simulink model "AMR_main_23b"  (R2024a)
settings: configuration reference "Configuration" (kept outside this file)
model workspace (MAT data in the model file):
  RTK_health_condition = 30
  mdlWSDbList = ["C:\Users\matlab.cut\Desktop\AMR\canbus_files\tramontina_database_nvidia.dbc" "C:\Users\matlab.cut\Desktop\AMR\canbus_files\tramontina_database_sick_modbus.dbc" "C:\Users\matlab.cut\Desktop\AMR\canbus_files\tramontina_database_xsens.dbc" "tramontina_database_curtis.dbc"]
undefined symbols (not defined in the file or in its folder): Down, Pull
libraries: speedgoatlib_IO60X_IO69X x17, tramontina_database_nvidialib x11, tramontina_database_curtislib x7, tramontina_database_xsenslib x4, tramontina_database_moboticlib x4, speedgoatlib_IO691 x3, canmsglib x2, slrealtimeseriallib x2, etargetslib x1, tramontina_database_sick_modbuslib x1
(part 1 of 2)
settings Model: DataDictionary=configuration_dictionary.sldd  Creator=matlab.cut  LastModifiedBy=rodri
settings ConfigSetRef: SourceName=Configuration

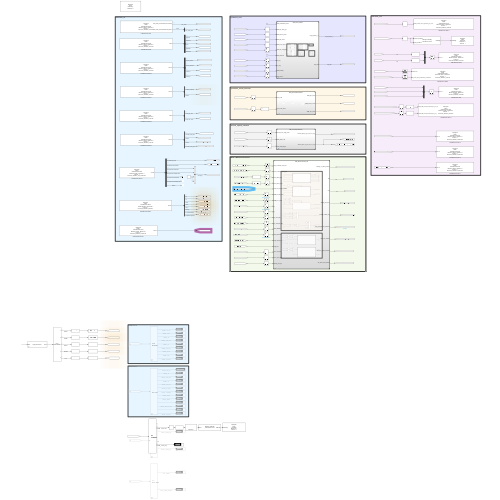
[thumbnail: Simulink's stored preview of the top-level diagram]
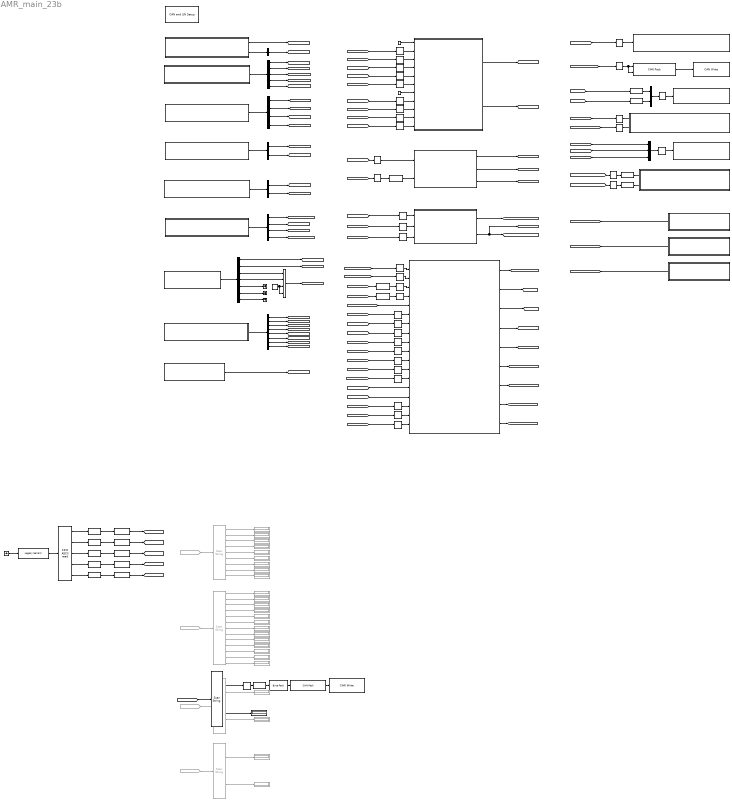
== system AMR_main_23b ==
  note: interface_in
  note: interface_out
  note: guidance_unit
  note: operation_mode_selector
  note: vehicle_speed_readout
  note: MCU - MotorControlUnit
  note: GPGGA Parser
  note: GPRMC Parser
  ASCII to String{,1..4} (5 alike) : ASCIIToString
  Bus Creator2 : BusCreator  Inputs=2
  Bus Creator3 : BusCreator  Inputs=3
  Bus Selector : BusSelector  OutputSignals=ID113_LongLat.latitude,ID113_LongLat.longitude,ID34_EulerAngles.yaw,ID17_StatusWord.GNSSfix,ID17_StatusWord.RtkStatus
  Bus Selector1 : BusSelector  OutputSignals=ID288_mobotic_feedback_pos.position_feedback,ID288_mobotic_feedback_pos.MessageStatus.Status
  Bus Selector2 : BusSelector  OutputSignals=ID422_curtis_feedback_message_left.motor_rpm_left,ID423_curtis_feedback_message_right.motor_rpm_right
  Bus Selector3 : BusSelector  OutputSignals=ID370_outdoor_scanner_PosX.X,ID371_outdoor_scanner_PosY.Y,ID372_outdoor_scanner_Yaw_Status.Yaw,ID373_outdoor_scanner_Odometer_Vel.velX,ID373_outdoor_scanner_Odometer_Vel.velY,ID373_outdoor_scanner_Odometer_Vel.velAng,ID372_outdoor_scanner_Yaw_Status.LocalizationStatus,ID372_outdoor_scanner_Yaw_Status.MapMatchingStatus
  Bus Selector4 : BusSelector  OutputSignals=Status  OutputAsBus=on
  Bus Selector5 : BusSelector  OutputSignals=ID368_joystick_axes.joystick_throttle,ID368_joystick_axes.joystick_direction,ID369_joystick_buttons.button_5,ID369_joystick_buttons.button_6
  Bus Selector6 : BusSelector  OutputSignals=ID1830_controller_status_left.controller_mode_left,ID1830_controller_status_left.MessageStatus.Status,ID1831_controller_status_right.MessageStatus.Status,ID1831_controller_status_right.controller_mode_right
  Bus Selector7 : BusSelector  OutputSignals=ID341_read_from_flexisoft.AuxEmEmergencia,ID341_read_from_flexisoft.AuxScannerInterrompido,ID341_read_from_flexisoft.EmergenciaFrontalDireita,ID341_read_from_flexisoft.EmergenciaFrontalEsquerda,ID341_read_from_flexisoft.EmergenciaTraseiraDireita,ID341_read_from_flexisoft.EmergenciaTraseiraEsquerda,ID341_read_from_flexisoft.MessageStatus.Status
  Byte Pack : etargetslib/Byte Pack  datatypes={'double'}  byteAlign=1
  CAN DB Parser Read : Subsystem
      settings: OpenFcn=sg_can.OpenFcnRead;
      mask Help: eval('sg.utils.help.show(''io_main/refentry_ref_can_ofa_parsing_read'');')
      mask Display: disp('Speedgoat\nIO691\nCAN DB Parser Read\nModule ID: IO691 - Module ID 1\nChannel:  1\ntramontina_database_xsens.dbc ');
  "CAN DB Parser Read " : Subsystem
      settings: OpenFcn=sg_can.OpenFcnRead;
      mask Help: eval('sg.utils.help.show(''io_main/refentry_ref_can_ofa_parsing_read'');')
      mask Display: disp('Speedgoat\nIO691\nCAN DB Parser Read\nModule ID: IO691 - Module ID 1\nChannel:  1\ntramontina_database_nvidia.dbc ');
  CAN DB Parser Read 1 : Subsystem
      settings: OpenFcn=sg_can.OpenFcnRead;
      mask Help: eval('sg.utils.help.show(''io_main/refentry_ref_can_ofa_parsing_read'');')
      mask Display: disp('Speedgoat\nIO691\nCAN DB Parser Read\nModule ID: IO691 - Module ID 1\nChannel:  1\ntramontina_database_nvidia.dbc ');
  CAN DB Parser Read 2 : Subsystem
      settings: OpenFcn=sg_can.OpenFcnRead;
      mask Help: eval('sg.utils.help.show(''io_main/refentry_ref_can_ofa_parsing_read'');')
      mask Display: disp('Speedgoat\nIO691\nCAN DB Parser Read\nModule ID: IO691 - Module ID 1\nChannel:  1\ntramontina_database_curtis.dbc ');
  CAN DB Parser Read 3 : Subsystem
      settings: OpenFcn=sg_can.OpenFcnRead;
      mask Help: eval('sg.utils.help.show(''io_main/refentry_ref_can_ofa_parsing_read'');')
      mask Display: disp('Speedgoat\nIO691\nCAN DB Parser Read\nModule ID: IO691 - Module ID 1\nChannel:  1\ntramontina_database_curtis.dbc ');
  CAN DB Parser Read 4 : Subsystem
      settings: OpenFcn=sg_can.OpenFcnRead;
      mask Help: eval('sg.utils.help.show(''io_main/refentry_ref_can_ofa_parsing_read'');')
      mask Display: disp('Speedgoat\nIO691\nCAN DB Parser Read\nModule ID: IO691 - Module ID 1\nChannel:  1\ntramontina_database_sick_modbus.dbc ');
  CAN DB Parser Read 5 : Subsystem
      settings: OpenFcn=sg_can.OpenFcnRead;
      mask Help: eval('sg.utils.help.show(''io_main/refentry_ref_can_ofa_parsing_read'');')
      mask Display: disp('Speedgoat\nIO691\nCAN DB Parser Read\nModule ID: IO691 - Module ID 1\nChannel:  1\ntramontina_database_nvidia.dbc ');
  CAN DB Parser Read 6 : Subsystem
      settings: OpenFcn=sg_can.OpenFcnRead;
      mask Help: eval('sg.utils.help.show(''io_main/refentry_ref_can_ofa_parsing_read'');')
      mask Display: disp('Speedgoat\nIO691\nCAN DB Parser Read\nModule ID: IO691 - Module ID 1\nChannel:  1\ntramontina_database_nvidia.dbc ');
  CAN DB Parser Read 7 : Subsystem
      settings: OpenFcn=sg_can.OpenFcnRead;
      mask Help: eval('sg.utils.help.show(''io_main/refentry_ref_can_ofa_parsing_read'');')
      mask Display: disp('Speedgoat\nIO691\nCAN DB Parser Read\nModule ID: IO691 - Module ID 1\nChannel:  1\ntramontina_database_mobotic.dbc ');
  "CAN DB Parser Write " : Subsystem
      settings: OpenFcn=sg_can.OpenFcnWrite;
      mask Help: eval('sg.utils.help.show(''io_main/refentry_ref_can_ofa_parsing_write'');')
      mask Display: disp('Speedgoat\nIO691\nCAN DB Parser Write\nModule ID: IO691 - Module ID 1\nChannel:  1\ntramontina_database_nvidia.dbc ');
  CAN DB Parser Write 1 : Subsystem
      settings: OpenFcn=sg_can.OpenFcnWrite;
      mask Help: eval('sg.utils.help.show(''io_main/refentry_ref_can_ofa_parsing_write'');')
      mask Display: disp('Speedgoat\nIO691\nCAN DB Parser Write\nModule ID: IO691 - Module ID 1\nChannel:  1\ntramontina_database_nvidia.dbc ');
  CAN DB Parser Write 2 : Subsystem
      settings: OpenFcn=sg_can.OpenFcnWrite;
      mask Help: eval('sg.utils.help.show(''io_main/refentry_ref_can_ofa_parsing_write'');')
      mask Display: disp('Speedgoat\nIO691\nCAN DB Parser Write\nModule ID: IO691 - Module ID 1\nChannel:  1\ntramontina_database_curtis.dbc ');
  CAN DB Parser Write 3 : Subsystem
      settings: OpenFcn=sg_can.OpenFcnWrite;
      mask Help: eval('sg.utils.help.show(''io_main/refentry_ref_can_ofa_parsing_write'');')
      mask Display: disp('Speedgoat\nIO691\nCAN DB Parser Write\nModule ID: IO691 - Module ID 1\nChannel:  1\ntramontina_database_curtis.dbc ');
  CAN DB Parser Write 4 : Subsystem
      settings: OpenFcn=sg_can.OpenFcnWrite;
      mask Help: eval('sg.utils.help.show(''io_main/refentry_ref_can_ofa_parsing_write'');')
      mask Display: disp('Speedgoat\nIO691\nCAN DB Parser Write\nModule ID: IO691 - Module ID 1\nChannel:  1\ntramontina_database_mobotic.dbc ');
  CAN DB Parser Write 5 : Subsystem
      settings: OpenFcn=sg_can.OpenFcnWrite;
      mask Help: eval('sg.utils.help.show(''io_main/refentry_ref_can_ofa_parsing_write'');')
      mask Display: disp('Speedgoat\nIO691\nCAN DB Parser Write\nModule ID: IO691 - Module ID 1\nChannel:  1\ntramontina_database_nvidia.dbc ');
  CAN DB Parser Write 6 : Subsystem
      settings: OpenFcn=sg_can.OpenFcnWrite;
      mask Help: eval('sg.utils.help.show(''io_main/refentry_ref_can_ofa_parsing_write'');')
      mask Display: disp('Speedgoat\nIO691\nCAN DB Parser Write\nModule ID: IO691 - Module ID 1\nChannel:  1\ntramontina_database_mobotic.dbc ');
  CAN DB Parser Write 7 : Subsystem
      settings: OpenFcn=sg_can.OpenFcnWrite;
      mask Help: eval('sg.utils.help.show(''io_main/refentry_ref_can_ofa_parsing_write'');')
      mask Display: disp('Speedgoat\nIO691\nCAN DB Parser Write\nModule ID: IO691 - Module ID 1\nChannel:  1\ntramontina_database_mobotic.dbc ');
  CAN Pack : canmsglib/CAN Pack  MsgList=(none)  MsgName=CAN Msg  MsgIDType=Standard (11-bit identifier)  MsgIdentifier=0x123  MsgLength=8  Remote=off  ApplyMinMax=off  BusOutput=on  SignalInfo={}
      settings: LibrarySourceBlock=embeddedtargetslib/Host Communication/CAN Pack  DataFormat=raw data
  CAN Pack2 : canmsglib/CAN Pack  MsgList=(none)  MsgName=CAN Msg  MsgIDType=Standard (11-bit identifier)  MsgIdentifier=0x120  MsgLength=8  Remote=off  ApplyMinMax=off  BusOutput=on  SignalInfo={ 'position_feedback', '0', '32', 'LE', 'signed', 'Standard', '0', '1', '0', '-inf', 'inf'; 'pulse_feedback', '32', '32', 'LE', 'signed', 'Standard', '0', '1', '0', '-Inf', 'Inf' }
      settings: DataFormat=manually specified signals
  CAN Write 1 : speedgoatlib_IO691/CAN Write   moduleType=IO691  id=1  channel=1  canType=CAN (HS)  messageType=CAN (HS)  useBusIn=on  numOfMsg=1  enableInput=off  enableStatusPort=off  ts=100e-3  initValues=[691 1 0.1 0 1 1 0 1 0 1]
      settings: SourceProductName=IO691
  CAN Write 2 : speedgoatlib_IO691/CAN Write   moduleType=IO691  id=1  channel=1  canType=CAN (HS)  messageType=CAN (HS)  useBusIn=on  numOfMsg=1  enableInput=off  enableStatusPort=off  ts=20e-3  initValues=[691 1 0.02 0 1 1 0 1 0 1]
      settings: SourceProductName=IO691
  "CAN and LIN Setup " : speedgoatlib_IO691/CAN and LIN Setup   moduleInitValues="[691    1    1   -1   -1]"  id=1  moduleType=IO691  pciSlot=-1  canChn1=CAN (HS)  canChn2=Disabled  canChn3=Disabled  canChn4=Disabled  linChn1=Disabled  linChn2=Disabled  canInitStructArray=[]  canTermStructArray=[]  gpioChnx=Disabled  canChn1InitValues="[2   2   8   1  16   3  19   2   2   5   2   0]"  arbBdrChn1=500 kBaud  clockDividerChn1=Enable  arbManBdrChn1=[8,1,16,3]  fdBdrChn1=5.0 MBaud  fdManBdrChn1=[2,2,5,2]  termResistor1=off  canChn2InitValues="[1   0   2   8  31   8  19   2   2   5   2   0]"  arbBdrChn2=1.0 MBaud  clockDividerChn2=Enable  arbManBdrChn2=[2,8,31,8]  fdBdrChn2=5.0 MBaud  fdManBdrChn2=[2,2,5,2]  termResistor2=off  canChn3InitValues="[1   0   2   8  31   8  19   2   2   5   2   0]"  arbBdrChn3=1.0 MBaud  clockDividerChn3=Enable  arbManBdrChn3=[2,8,31,8]  fdBdrChn3=5.0 MBaud  fdManBdrChn3=[2,2,5,2]  termResistor3=off  canChn4InitValues="[1   0   2   8  31   8  19   2   2   5   2   0]"  arbBdrChn4=1.0 MBaud  clockDividerChn4=Enable  arbManBdrChn4=[2,8,31,8]  fdBdrChn4=5.0 MBaud  fdManBdrChn4=[2,2,5,2]  termResistor4=off  linChn1InitValues="[0  9600]"  linBtrChn1=9600  linChn2InitValues="[0  9600]"  linBtrChn2=9600  doInitTermStruct="[0  5  0  0  0]"  parDoChannels=[1 2]  parDoVoltage=5  parDoInitValues=0  parDoReset=1  parNumOfDoS=0  parDiChannels=[3 4]  parDiVoltage=5  parDiPull=Pull-Down
      settings: LibrarySourceBlock=speedgoatlib_IO602_IO691/CAN and LIN Setup
  Cast{,6..9} (5 alike) : DataTypeConversion  OutDataTypeStr=uint8  SaturateOnIntegerOverflow=off  RndMeth=Floor
  Cast1 : DataTypeConversion  OutDataTypeStr=boolean  SaturateOnIntegerOverflow=off  RndMeth=Floor
  Cast10 : DataTypeConversion  OutDataTypeStr=double  SaturateOnIntegerOverflow=off  RndMeth=Floor
  Cast11 : DataTypeConversion  OutDataTypeStr=double  SaturateOnIntegerOverflow=off  RndMeth=Floor
  Cast12 : DataTypeConversion  OutDataTypeStr=double  SaturateOnIntegerOverflow=off  RndMeth=Floor
  Cast2 : DataTypeConversion  OutDataTypeStr=single  SaturateOnIntegerOverflow=off  RndMeth=Floor
  Cast3 : DataTypeConversion  OutDataTypeStr=single  SaturateOnIntegerOverflow=off  RndMeth=Floor
  Cast4 : DataTypeConversion  OutDataTypeStr=boolean  SaturateOnIntegerOverflow=off  RndMeth=Floor
  Cast5 : DataTypeConversion  OutDataTypeStr=boolean  SaturateOnIntegerOverflow=off  RndMeth=Floor
  Display{2..4,6,8..12,14..18,20..31} (26 alike) : Display  Commented=on
  Display5 : Display
  FIFO ASCII read : slrealtimeseriallib/FIFO ASCII read  header={'$GPGGA', '$GPRMC','$HEHDT','$HCHDM','$PTCF'}  term=[13 10]  hold=Hold last output if no new data  enable=off  maxsize=1024  outputtype=8 bit uint null terminated  sampletime=-1
  From18 : From  Commented=on  GotoTag=PTCF_decode
  From22 : From  Commented=on  GotoTag=GPRMC_decode
  From23 : From  Commented=on  GotoTag=GPGGA_decode
  From30 : From  Commented=on  GotoTag=HEHDT_decode
  Ground3 : Ground
  Legacy Serial F2 : slrealtimeseriallib/Mainboard/Legacy Serial F  port=Legacy Serial Port 1  baud=115200  width=8  nstop=1  parity=None  ctsmode=off  fifosize=1024  idtype=8 bit uint null terminated  sampletime=10e-3
  Model : ModelReference  ModelNameDialog=deployAGV_stateflow.slx  SimulationMode=Normal  ModelReferenceVersion=3.4
  Model1 : ModelReference  ModelNameDialog=AMR_OperationModeSelector.slx  SimulationMode=Normal  ModelReferenceVersion=2.0
  Model3 : ModelReference  ModelNameDialog=AMR_VehicleSpeedReadout.slx  SimulationMode=Normal  ModelReferenceVersion=2.0
  Model4 : ModelReference  ModelNameDialog=AMR_MotorControlUnit_23b.slx  SimulationMode=Normal  ModelReferenceVersion=2.3
  OR : Logic  Operator=OR  Inputs=4  AllPortsSameDT=off  OutDataTypeStr=boolean
  Rate Transition{,1..10,13..16,22..24,26,28..30,32..44} (35 alike) : RateTransition
  Rate Transition11 : RateTransition  OutPortSampleTimeOpt=Inherit
  Rate Transition12 : RateTransition  Deterministic=off
  Rate Transition21 : RateTransition  OutPortSampleTimeOpt=Inherit
  String to Double : ScanString  Commented=on  Format="\"$GPRMC,%f,%c,%f,%c,%f,%c,%f,,%d,,,%s\""
  String to Double1 : ScanString  Commented=on  Format="\"$GPGGA,%f,%f,%c,%f,%c,%d,%d,%f,%f,%c,%g,%c,,%f\""
  String to Double2 : ScanString  Commented=on  Format="\"$HEHDT,%f,%c\""
  String to Double3 : ScanString  Format="\"$HCHDM,%f,%c\""
  String to Double4 : ScanString  Commented=on  Format="\"$PTCF,%f,%c\""
  Terminator : Terminator
  Terminator1 : Terminator
  Terminator2 : Terminator
  Zero : Constant  Value=0  OutDataTypeStr=Inherit: Inherit via back propagation
  Zero1 : Constant  Value=0  OutDataTypeStr=Inherit: Inherit via back propagation
  Zero2 : Constant  Value=0  OutDataTypeStr=Inherit: Inherit via back propagation
  wires:
  Bus Selector7/2 -> [scanner_blocked]  "<AuxScannerInterrompido>"
  Bus Selector4/1 -> [oper_mode_status]  "oper_mode_status"
  Bus Selector6/4 -> [curtis_controller_mode_right]  "<controller_mode_right>"
  Bus Selector7/3 -> OR/1  "<EmergenciaFrontalDireita>"
  "CAN DB Parser Read "/1(ID343_AMR_OperationMode.OperationMode) -> [oper_mode]  "oper_mode"
  Bus Selector1/2 -> [steering_unit_status]  "<Status>"
  Bus Selector/1 -> [lat_deg]  "<latitude>"
  Bus Selector5/3 -> [joy_boost_flag]  "<button_5>"
  CAN DB Parser Read/1(CAN Rx) -> Bus Selector/1
  Bus Selector/5 -> [GPS_RTKstatus]  "<RtkStatus>"
  Bus Selector5/1 -> [xj]  "<joystick_throttle>"
  Zero/1 -> OR/3, OR/4
  Bus Selector/4 -> [GPS_GNSSfix]  "<GNSSfix>"
  Bus Selector6/2 -> [curtis_status_left]  "<Status>"
  Bus Selector/2 -> [lon_deg]  "<longitude>"
  Bus Selector7/6 -> Terminator1/1  "<EmergenciaTraseiraEsquerda>"
  "CAN DB Parser Read "/2(ID343_AMR_OperationMode.MessageStatus) -> Bus Selector4/1  "status"
  Bus Selector7/4 -> OR/2  "<EmergenciaFrontalEsquerda>"
  Bus Selector7/7 -> Terminator/1  "<Status>"
  Bus Selector5/2 -> [yj]  "<joystick_direction>"
  CAN DB Parser Read 2/1(CAN Rx) -> Bus Selector2/1
  Bus Selector2/2 -> [motor_rpm_right]  "<motor_rpm_right>"
  CAN DB Parser Read 4/1(CAN Rx) -> Bus Selector7/1
  CAN DB Parser Read 3/1(CAN Rx) -> Bus Selector6/1
  Bus Selector6/1 -> [curtis_controller_mode_left]  "<controller_mode_left>"
  Bus Selector2/1 -> [motor_rpm_left]  "<motor_rpm_left>"
  Bus Selector6/3 -> [curtis_status_right]  "<Status>"
  Bus Selector1/1 -> [steering_unit_pos]  "<position_feedback>"
  CAN DB Parser Read 5/1(CAN Rx) -> Bus Selector5/1
  Bus Selector/3 -> [AMR_heading]  "<yaw>"
  CAN DB Parser Read 1/1(CAN Rx) -> Bus Selector1/1
  OR/1 -> [emergency]  "emergency"
  Bus Selector5/4 -> [joy_maxspeed_flag]  "<button_6>"
  Bus Selector7/5 -> Terminator2/1  "<EmergenciaTraseiraDireita>"
  Bus Selector7/1 -> [interlock]  "<AuxEmEmergencia>"
  Rate Transition32/1 -> CAN DB Parser Write 5/1(ID289_mobotic_error_flag.steering_unit_error)
  Rate Transition28/1 -> Cast2/1
  [AMR_speed_to_CAN_m_per_sec] -> Rate Transition29/1
  [AMR_speed_to_CAN_m_per_min] -> Rate Transition28/1
  CAN Pack2/1 -> CAN Write 2/1
  Bus Creator2/1 -> Rate Transition15/1
  [rws] -> Cast11/1  "rws"
  Cast10/1 -> Bus Creator2/1
  Rate Transition6/1 -> CAN DB Parser Write 3/2(ID0_curtis_input_operational.pre_operational)
  Bus Creator3/1 -> Rate Transition12/1
  [steering_unit_error] -> Rate Transition32/1
  Rate Transition10/1 -> CAN Pack2/2, CAN Pack2/1
  Rate Transition29/1 -> Cast3/1
  [curtis_controller_into_operation] -> Rate Transition6/1
  [lws] -> Cast10/1  "lws"
  Cast11/1 -> Bus Creator2/2
  [steering_unit_theta_position] -> Rate Transition10/1
  [controller_enable_flag] -> Rate Transition24/1
  Rate Transition15/1 -> CAN DB Parser Write 2/1(CAN Tx)
  Rate Transition24/1 -> CAN DB Parser Write 3/1(Enable Input)
  [AMR_heading] -> Rate Transition39/1
  [lon_deg] -> Rate Transition36/1
  [AMR_manual_mode] -> Rate Transition30/1
  [interlock] -> Rate Transition44/1
  [emergency] -> Rate Transition43/1
  [scanner_blocked] -> Rate Transition42/1
  [lat_deg] -> Rate Transition35/1
  [AMR_speed] -> Rate Transition37/1
  Rate Transition44/1 -> Model/2
  Zero1/1 -> Model/1
  Rate Transition30/1 -> Model/3
  Model/1 -> [target_speed_m_s]  "target_speed_m_s"
  Model/2 -> [angle_diff]  "angle_diff"
  [oper_mode] -> Rate Transition/1
  Cast4/1 -> Model1/2
  Model1/1 -> [AMR_idle_mode]
  Model1/2 -> [AMR_manual_mode]
  Model1/3 -> [AMR_auto_mode]
  [xj] -> Rate Transition3/1
  [joy_boost_flag] -> Rate Transition5/1
  [curtis_controller_mode_left] -> Rate Transition21/1
  Rate Transition22/1 -> Model4/3
  [yj] -> Rate Transition4/1
  Rate Transition21/1 -> Model4/1
  Rate Transition23/1 -> Model4/4
  Rate Transition11/1 -> Model4/2
  [joy_maxspeed_flag] -> Rate Transition7/1
  [AMR_manual_mode] -> Rate Transition16/1
  [curtis_status_right] -> Cast1/1
  [curtis_status_left] -> Cast5/1
  [curtis_controller_mode_right] -> Rate Transition11/1
  [AMR_auto_mode] -> Rate Transition33/1
  [motor_rpm_right] -> Rate Transition41/1
  [steering_unit_pos] -> Rate Transition38/1
  [motor_rpm_left] -> Rate Transition40/1
  Model3/1 -> [AMR_speed_to_CAN_m_per_min]
  Model3/2 -> [AMR_speed_to_CAN_m_per_sec], [AMR_speed]
  Rate Transition38/1 -> Model3/1
  Rate Transition41/1 -> Model3/3
  Rate Transition40/1 -> Model3/2
  Model4/1 -> [steering_unit_theta_position]
  Model4/3 -> [rws]  "rws"
  Model4/2 -> [lws]  "lws"
  [GPS_GNSSfix] -> Rate Transition34/1
  [motor_rpm_left] -> Rate Transition26/1
  [motor_rpm_right] -> Rate Transition9/1
  [steering_unit_pos] -> Rate Transition14/1
  Model4/4 -> [steering_unit_error]
  Model4/5 -> [controller_enable_flag]
  Model4/6 -> [curtis_controller_into_operation]
  [GPS_RTKstatus] -> Rate Transition8/1
  Cast2/1 -> CAN DB Parser Write 1/1(ID290_AMR_vehicle_speed.speed_m_per_min)
  Cast3/1 -> CAN DB Parser Write 1/2(ID290_AMR_vehicle_speed.speed_m_per_s)
  [oper_mode_status] -> Rate Transition1/1
  [AMR_idle_mode] -> Bus Creator3/1
  [AMR_auto_mode] -> Bus Creator3/3
  [AMR_manual_mode] -> Bus Creator3/2
  Cast5/1 -> Rate Transition22/1
  Cast1/1 -> Rate Transition23/1
  Rate Transition12/1 -> "CAN DB Parser Write "/1(CAN Tx)
  Rate Transition/1 -> Model1/1
  Rate Transition1/1 -> Cast4/1
  CAN DB Parser Read 6/1(CAN Rx) -> Bus Selector3/1
  Bus Selector3/6 -> [sick_vel_ang]  "<velAng>"
  Bus Selector3/1 -> [sick_x]  "<X>"
  Bus Selector3/4 -> [sick_velx]  "<velX>"
  Bus Selector3/2 -> [sick_y]  "<Y>"
  Bus Selector3/3 -> [sick_yaw]  "<Yaw>"
  Bus Selector3/5 -> [sick_vely]  "<velY>"
  Bus Selector3/7 -> [sick_loc_status]  "<LocalizationStatus>"
  Bus Selector3/8 -> [sick_map_matching]  "<MapMatchingStatus>"
  Legacy Serial F2/1 -> FIFO ASCII read/1
  FIFO ASCII read/5 -> Cast6/1  "PTCF"
  From18/1 -> String to Double4/1
  Cast6/1 -> ASCII to String4/1
  String to Double4/2 -> Display30/1  "PTCF__heading_TrueNorth"
  ASCII to String3/1 -> [HCHDM_decode]
  String to Double4/1 -> Display31/1  "PTCF__heading"
  FIFO ASCII read/2 -> Cast/1  "GPRMC"
  String to Double/5 -> Display21/1  "GPRMC__lon"
  String to Double2/2 -> Display12/1  "HEHDT__heading_type"
  String to Double1/13 -> Display29/1  "GPGGA__checksum"
  ASCII to String4/1 -> [PTCF_decode]
  String to Double1/5 -> Display15/1  "GPGGA__east_west"
  String to Double1/10 -> Display28/1
  ASCII to String2/1 -> [GPGGA_decode]
  Cast9/1 -> ASCII to String3/1
  String to Double2/1 -> Display6/1  "HEHDT__heading_deg"
  FIFO ASCII read/3 -> Cast8/1  "HEHDT"
  String to Double/7 -> Display3/1  "GPRMC__speed"
  FIFO ASCII read/4 -> Cast9/1  "HCHDM"
  From23/1 -> String to Double1/1
  String to Double1/11 -> Display24/1  "GPGGA__mean_sea_level"
  String to Double1/1 -> Display14/1  "GPGGA__time_utc"
  String to Double/2 -> Display22/1  "GPRMC__status"
  FIFO ASCII read/1 -> Cast7/1  "GPGGA"
  [HCHDM_decode] -> String to Double3/1
  Cast/1 -> ASCII to String/1
  String to Double1/8 -> Display26/1  "GPGGA__HDOP"
  String to Double/3 -> Display23/1  "GPRMC__lat"
  String to Double1/7 -> Display18/1  "GPGGA__#_satellites"
  String to Double/6 -> Display2/1  "GPRMC__east_west"
  From22/1 -> String to Double/1
  String to Double/4 -> Display11/1  "GPRMC__north_south"
  Cast8/1 -> ASCII to String1/1
  String to Double1/12 -> Display25/1
  String to Double/8 -> Display4/1  "GPRMC__date"
  ASCII to String/1 -> [GPRMC_decode]
  String to Double/1 -> Display20/1  "GPRMC__time_utc"
  String to Double/9 -> Display8/1  "GPRMC__checksum"
  ASCII to String1/1 -> [HEHDT_decode]
  String to Double1/6 -> Display10/1  "GPGGA__fix_quality"
  String to Double1/2 -> Display16/1  "GPGGA__lat"
  From30/1 -> String to Double2/1
  String to Double3/1 -> Rate Transition2/1  "HCHDM__heading_deg"
  String to Double1/3 -> Display17/1  "GPGGA__north_south"
  String to Double1/4 -> Display9/1  "GPGGA__lon"
  String to Double3/2 -> Display5/1  "HCHDM__heading_mag"
  Ground3/1 -> Legacy Serial F2/1
  String to Double1/9 -> Display27/1  "GPGGA__altitude"
  Cast7/1 -> ASCII to String2/1
  Rate Transition2/1 -> Cast12/1
  Cast12/1 -> Byte Pack/1
  CAN Pack/1 -> CAN Write 1/1
  Rate Transition39/1 -> Model/10
  Rate Transition37/1 -> Model/11
  Zero2/1 -> Model/7
  Rate Transition43/1 -> Model/6
  Rate Transition42/1 -> Model/5
  [AMR_idle_mode] -> Rate Transition13/1
  Rate Transition35/1 -> Model/8
  Rate Transition36/1 -> Model/9
  Rate Transition13/1 -> Model/4
  Byte Pack/1 -> CAN Pack/1
  CAN DB Parser Read 7/1(CAN Rx) -> [read_error_register_CANRx]
  [read_error_register_CANRx] -> Model4/5
  Rate Transition16/1 -> Model4/6
  Rate Transition33/1 -> Model4/7
  Rate Transition3/1 -> Model4/8
  Rate Transition4/1 -> Model4/9
  Rate Transition5/1 -> Model4/10
  Rate Transition7/1 -> Model4/11
  Rate Transition34/1 -> Model4/12
  Rate Transition8/1 -> Model4/13
  [target_speed_m_s] -> Model4/14
  [angle_diff] -> Model4/15
  Rate Transition26/1 -> Model4/16
  Rate Transition9/1 -> Model4/17
  Rate Transition14/1 -> Model4/18
  Model4/7 -> [clear_error_CANTx]
  Model4/8 -> [read_error_request_CANTx]
  Model4/9 -> [set_sevice_state_CANTx]
  [clear_error_CANTx] -> CAN DB Parser Write 6/1(CAN Tx)
  [read_error_request_CANTx] -> CAN DB Parser Write 4/1(CAN Tx)
  [set_sevice_state_CANTx] -> CAN DB Parser Write 7/1(CAN Tx)

== system AMR_main_23b/CAN DB Parser Read ==
  ReadSubsystem : Subsystem
  UnpackSubsystem : Subsystem
  CAN Rx : Outport
  wires:
  ReadSubsystem/1(Raw_Rx) -> UnpackSubsystem/1(Unpack_In)
  ReadSubsystem/2(Status_Rx) -> UnpackSubsystem/2(Status Inport)
  UnpackSubsystem/1(Unpack_Out) -> CAN Rx/1

== system AMR_main_23b/CAN DB Parser Read  ==
  ReadSubsystem : Subsystem
  SelectSignal_1_1 : BusSelector  OutputSignals=ID343_AMR_OperationMode.OperationMode
  SelectStatus_1 : BusSelector  OutputSignals=ID343_AMR_OperationMode.MessageStatus
  UnpackSubsystem : Subsystem
  ID343_AMR_OperationMode.OperationMode : Outport
  ID343_AMR_OperationMode.MessageStatus : Outport  Port=2
  wires:
  ReadSubsystem/1(Raw_Rx) -> UnpackSubsystem/1(Unpack_In)
  ReadSubsystem/2(Status_Rx) -> UnpackSubsystem/2(Status Inport)
  UnpackSubsystem/1(Unpack_Out) -> SelectSignal_1_1/1, SelectStatus_1/1
  SelectSignal_1_1/1 -> ID343_AMR_OperationMode.OperationMode/1  "<OperationMode>"
  SelectStatus_1/1 -> ID343_AMR_OperationMode.MessageStatus/1  "<MessageStatus>"

== system AMR_main_23b/CAN DB Parser Read 1 ==
  ReadSubsystem : Subsystem
  UnpackSubsystem : Subsystem
  CAN Rx : Outport
  wires:
  ReadSubsystem/1(Raw_Rx) -> UnpackSubsystem/1(Unpack_In)
  ReadSubsystem/2(Status_Rx) -> UnpackSubsystem/2(Status Inport)
  UnpackSubsystem/1(Unpack_Out) -> CAN Rx/1

== system AMR_main_23b/CAN DB Parser Read 2 ==
  ReadSubsystem : Subsystem
  UnpackSubsystem : Subsystem
  CAN Rx : Outport
  wires:
  ReadSubsystem/1(Raw_Rx) -> UnpackSubsystem/1(Unpack_In)
  ReadSubsystem/2(Status_Rx) -> UnpackSubsystem/2(Status Inport)
  UnpackSubsystem/1(Unpack_Out) -> CAN Rx/1

== system AMR_main_23b/CAN DB Parser Read 3 ==
  ReadSubsystem : Subsystem
  UnpackSubsystem : Subsystem
  CAN Rx : Outport
  wires:
  ReadSubsystem/1(Raw_Rx) -> UnpackSubsystem/1(Unpack_In)
  ReadSubsystem/2(Status_Rx) -> UnpackSubsystem/2(Status Inport)
  UnpackSubsystem/1(Unpack_Out) -> CAN Rx/1

== system AMR_main_23b/CAN DB Parser Read 4 ==
  ReadSubsystem : Subsystem
  UnpackSubsystem : Subsystem
  CAN Rx : Outport
  wires:
  ReadSubsystem/1(Raw_Rx) -> UnpackSubsystem/1(Unpack_In)
  ReadSubsystem/2(Status_Rx) -> UnpackSubsystem/2(Status Inport)
  UnpackSubsystem/1(Unpack_Out) -> CAN Rx/1

== system AMR_main_23b/CAN DB Parser Read 5 ==
  ReadSubsystem : Subsystem
  UnpackSubsystem : Subsystem
  CAN Rx : Outport
  wires:
  ReadSubsystem/1(Raw_Rx) -> UnpackSubsystem/1(Unpack_In)
  ReadSubsystem/2(Status_Rx) -> UnpackSubsystem/2(Status Inport)
  UnpackSubsystem/1(Unpack_Out) -> CAN Rx/1

== system AMR_main_23b/CAN DB Parser Read 6 ==
  ReadSubsystem : Subsystem
  UnpackSubsystem : Subsystem
  CAN Rx : Outport
  wires:
  ReadSubsystem/1(Raw_Rx) -> UnpackSubsystem/1(Unpack_In)
  ReadSubsystem/2(Status_Rx) -> UnpackSubsystem/2(Status Inport)
  UnpackSubsystem/1(Unpack_Out) -> CAN Rx/1

== system AMR_main_23b/CAN DB Parser Read 7 ==
  ReadSubsystem : Subsystem
  UnpackSubsystem : Subsystem
  CAN Rx : Outport
  wires:
  ReadSubsystem/1(Raw_Rx) -> UnpackSubsystem/1(Unpack_In)
  ReadSubsystem/2(Status_Rx) -> UnpackSubsystem/2(Status Inport)
  UnpackSubsystem/1(Unpack_Out) -> CAN Rx/1

== system AMR_main_23b/CAN DB Parser Write  ==
  CAN Tx : Inport
  BusMapping : Subsystem
  CANWrite : speedgoatlib_IO60X_IO69X/CAN/CAN Write   moduleType=IO691  id=1  channel=1  canType=CAN (HS)  messageType=CAN (HS)  useBusIn=on  numOfMsg=1  enableInput=on  enableStatusPort=off  ts=500e-3  initValues=[691 1 0.5 0 1 1 0 1 1 1]
  Convert2BusArray : Subsystem
  Enable All : Constant  OutDataTypeStr=boolean
  PackSubsystem : Subsystem
  Product : Product  OutDataTypeStr=uint32
  TxControl : Constant  Value=[1]  OutDataTypeStr=uint32
  wires:
  PackSubsystem/1(PackOut) -> Convert2BusArray/1(InBus)
  Convert2BusArray/1(BusArrayOut) -> CANWrite/2
  Product/1 -> CANWrite/1
  TxControl/1 -> Product/2
  Enable All/1 -> Product/1
  CAN Tx/1 -> BusMapping/1(InBus)
  BusMapping/1(OutBus) -> PackSubsystem/1(PackIn)

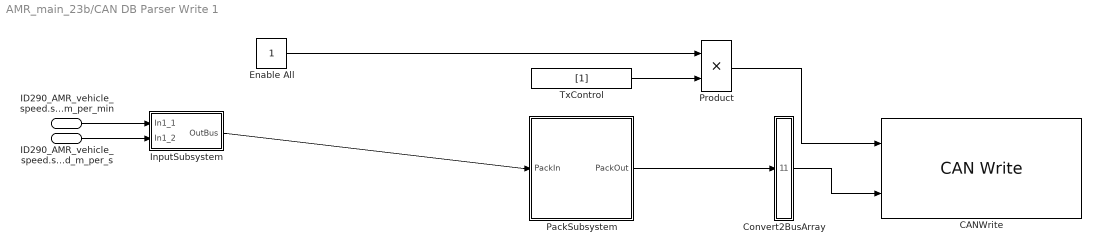
== system AMR_main_23b/CAN DB Parser Write 1 ==
  ID290_AMR_vehicle_speed.speed_m_per_min : Inport
  ID290_AMR_vehicle_speed.speed_m_per_s : Inport  Port=2
  CANWrite : speedgoatlib_IO60X_IO69X/CAN/CAN Write   moduleType=IO691  id=1  channel=1  canType=CAN (HS)  messageType=CAN (HS)  useBusIn=on  numOfMsg=1  enableInput=on  enableStatusPort=off  ts=50e-3  initValues=[691 1 0.05 0 1 1 0 1 1 1]
  Convert2BusArray : Subsystem
  Enable All : Constant  OutDataTypeStr=boolean
  InputSubsystem : Subsystem
  PackSubsystem : Subsystem
  Product : Product  OutDataTypeStr=uint32
  TxControl : Constant  Value=[1]  OutDataTypeStr=uint32
  wires:
  PackSubsystem/1(PackOut) -> Convert2BusArray/1(InBus)
  Convert2BusArray/1(BusArrayOut) -> CANWrite/2
  Product/1 -> CANWrite/1
  TxControl/1 -> Product/2
  Enable All/1 -> Product/1
  ID290_AMR_vehicle_speed.speed_m_per_min/1 -> InputSubsystem/1(In1_1)
  ID290_AMR_vehicle_speed.speed_m_per_s/1 -> InputSubsystem/2(In1_2)
  InputSubsystem/1(OutBus) -> PackSubsystem/1(PackIn)

== system AMR_main_23b/CAN DB Parser Write 2 ==
  CAN Tx : Inport
  BusMapping : Subsystem
  CANWrite : speedgoatlib_IO60X_IO69X/CAN/CAN Write   moduleType=IO691  id=1  channel=1  canType=CAN (HS)  messageType=CAN (HS)  useBusIn=on  numOfMsg=2  enableInput=on  enableStatusPort=off  ts=10e-3  initValues=[691 1 0.01 0 1 1 0 2 1 1]
  Convert2BusArray : Subsystem
  Enable All : Constant  OutDataTypeStr=boolean
  PackSubsystem : Subsystem
  Product : Product  OutDataTypeStr=uint32
  TxControl : Constant  Value="[1  1]"  OutDataTypeStr=uint32
  wires:
  PackSubsystem/1(PackOut) -> Convert2BusArray/1(InBus)
  Convert2BusArray/1(BusArrayOut) -> CANWrite/2
  Product/1 -> CANWrite/1
  TxControl/1 -> Product/2
  Enable All/1 -> Product/1
  CAN Tx/1 -> BusMapping/1(InBus)
  BusMapping/1(OutBus) -> PackSubsystem/1(PackIn)

== system AMR_main_23b/CAN DB Parser Write 3 ==
  Enable Input : Inport  OutDataTypeStr=boolean
  ID0_curtis_input_operational.pre_operational : Inport  Port=2
  CANWrite : speedgoatlib_IO60X_IO69X/CAN/CAN Write   moduleType=IO691  id=1  channel=1  canType=CAN (HS)  messageType=CAN (HS)  useBusIn=on  numOfMsg=1  enableInput=on  enableStatusPort=off  ts=500e-3  initValues=[691 1 0.5 0 1 1 0 1 1 1]
  Convert2BusArray : Subsystem
  InputSubsystem : Subsystem
  PackSubsystem : Subsystem
  Product : Product  OutDataTypeStr=uint32
  TxControl : Constant  Value=[1]  OutDataTypeStr=uint32
  wires:
  PackSubsystem/1(PackOut) -> Convert2BusArray/1(InBus)
  Convert2BusArray/1(BusArrayOut) -> CANWrite/2
  Product/1 -> CANWrite/1
  TxControl/1 -> Product/2
  Enable Input/1 -> Product/1
  ID0_curtis_input_operational.pre_operational/1 -> InputSubsystem/1(In1_1)
  InputSubsystem/1(OutBus) -> PackSubsystem/1(PackIn)

== system AMR_main_23b/CAN DB Parser Write 4 ==
  CAN Tx : Inport
  BusMapping : Subsystem
  CANWrite : speedgoatlib_IO60X_IO69X/CAN/CAN Write   moduleType=IO691  id=1  channel=1  canType=CAN (HS)  messageType=CAN (HS)  useBusIn=on  numOfMsg=1  enableInput=on  enableStatusPort=off  ts=-1  initValues=[691 1 -1 0 1 1 0 1 1 1]
  Convert2BusArray : Subsystem
  Enable All : Constant  OutDataTypeStr=boolean
  PackSubsystem : Subsystem
  Product : Product  OutDataTypeStr=uint32
  TxControl : Constant  Value=[1]  OutDataTypeStr=uint32
  wires:
  PackSubsystem/1(PackOut) -> Convert2BusArray/1(InBus)
  Convert2BusArray/1(BusArrayOut) -> CANWrite/2
  Product/1 -> CANWrite/1
  TxControl/1 -> Product/2
  Enable All/1 -> Product/1
  CAN Tx/1 -> BusMapping/1(InBus)
  BusMapping/1(OutBus) -> PackSubsystem/1(PackIn)

== system AMR_main_23b/CAN DB Parser Write 5 ==
  ID289_mobotic_error_flag.steering_unit_error : Inport
  CANWrite : speedgoatlib_IO60X_IO69X/CAN/CAN Write   moduleType=IO691  id=1  channel=1  canType=CAN (HS)  messageType=CAN (HS)  useBusIn=on  numOfMsg=1  enableInput=on  enableStatusPort=off  ts=500e-3  initValues=[691 1 0.5 0 1 1 0 1 1 1]
  Convert2BusArray : Subsystem
  Enable All : Constant  OutDataTypeStr=boolean
  InputSubsystem : Subsystem
  PackSubsystem : Subsystem
  Product : Product  OutDataTypeStr=uint32
  TxControl : Constant  Value=[1]  OutDataTypeStr=uint32
  wires:
  PackSubsystem/1(PackOut) -> Convert2BusArray/1(InBus)
  Convert2BusArray/1(BusArrayOut) -> CANWrite/2
  Product/1 -> CANWrite/1
  TxControl/1 -> Product/2
  Enable All/1 -> Product/1
  ID289_mobotic_error_flag.steering_unit_error/1 -> InputSubsystem/1(In1_1)
  InputSubsystem/1(OutBus) -> PackSubsystem/1(PackIn)

== system AMR_main_23b/CAN DB Parser Write 6 ==
  CAN Tx : Inport
  BusMapping : Subsystem
  CANWrite : speedgoatlib_IO60X_IO69X/CAN/CAN Write   moduleType=IO691  id=1  channel=1  canType=CAN (HS)  messageType=CAN (HS)  useBusIn=on  numOfMsg=1  enableInput=on  enableStatusPort=off  ts=-1  initValues=[691 1 -1 0 1 1 0 1 1 1]
  Convert2BusArray : Subsystem
  Enable All : Constant  OutDataTypeStr=boolean
  PackSubsystem : Subsystem
  Product : Product  OutDataTypeStr=uint32
  TxControl : Constant  Value=[1]  OutDataTypeStr=uint32
  wires:
  PackSubsystem/1(PackOut) -> Convert2BusArray/1(InBus)
  Convert2BusArray/1(BusArrayOut) -> CANWrite/2
  Product/1 -> CANWrite/1
  TxControl/1 -> Product/2
  Enable All/1 -> Product/1
  CAN Tx/1 -> BusMapping/1(InBus)
  BusMapping/1(OutBus) -> PackSubsystem/1(PackIn)

== system AMR_main_23b/CAN DB Parser Write 7 ==
  CAN Tx : Inport
  BusMapping : Subsystem
  CANWrite : speedgoatlib_IO60X_IO69X/CAN/CAN Write   moduleType=IO691  id=1  channel=1  canType=CAN (HS)  messageType=CAN (HS)  useBusIn=on  numOfMsg=1  enableInput=on  enableStatusPort=off  ts=-1  initValues=[691 1 -1 0 1 1 0 1 1 1]
  Convert2BusArray : Subsystem
  Enable All : Constant  OutDataTypeStr=boolean
  PackSubsystem : Subsystem
  Product : Product  OutDataTypeStr=uint32
  TxControl : Constant  Value=[1]  OutDataTypeStr=uint32
  wires:
  PackSubsystem/1(PackOut) -> Convert2BusArray/1(InBus)
  Convert2BusArray/1(BusArrayOut) -> CANWrite/2
  Product/1 -> CANWrite/1
  TxControl/1 -> Product/2
  Enable All/1 -> Product/1
  CAN Tx/1 -> BusMapping/1(InBus)
  BusMapping/1(OutBus) -> PackSubsystem/1(PackIn)

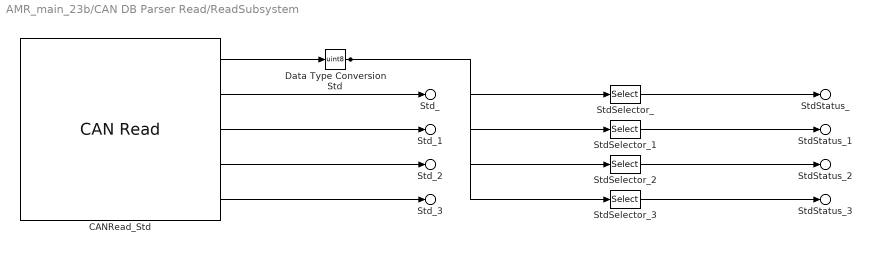
== system AMR_main_23b/CAN DB Parser Read/ReadSubsystem ==
  CANRead_Std : speedgoatlib_IO60X_IO69X/CAN/CAN Read   moduleType=IO691  id=1  channel=1  canType=CAN (HS)  messageType=CAN (HS)  useBusOut=on  HasMulRead=Specify by IDs  MsgIDlist="[17   34  113  118]"  isEFF=off  LabelInHex=off  enableInput=off  initValues=[691 1 0.005 0 1 1 0 1 2 0 4 17 34 113 118]  ts=5e-3
  Data Type ConversionStd : DataTypeConversion  OutDataTypeStr=uint8  SaturateOnIntegerOverflow=off  RndMeth=Floor
  StdSelector_ : Selector  IndexOptions=Index vector (dialog)  Indices=1  OutputSizes=1
  StdSelector_1 : Selector  IndexOptions=Index vector (dialog)  Indices=2  OutputSizes=1
  StdSelector_2 : Selector  IndexOptions=Index vector (dialog)  Indices=3  OutputSizes=1
  StdSelector_3 : Selector  IndexOptions=Index vector (dialog)  Indices=4  OutputSizes=1
  Std_ : Outport  PortName=Raw_Rx  Element=Std.ID17
  Std_1 : Outport  PortName=Raw_Rx  Element=Std.ID34
  Std_2 : Outport  PortName=Raw_Rx  Element=Std.ID113
  Std_3 : Outport  PortName=Raw_Rx  Element=Std.ID118
  StdStatus_ : Outport  Port=2  PortName=Status_Rx  Element=Std.ID17
  StdStatus_1 : Outport  Port=2  PortName=Status_Rx  Element=Std.ID34
  StdStatus_2 : Outport  Port=2  PortName=Status_Rx  Element=Std.ID113
  StdStatus_3 : Outport  Port=2  PortName=Status_Rx  Element=Std.ID118
  wires:
  CANRead_Std/1 -> Data Type ConversionStd/1
  CANRead_Std/2 -> Std_/1
  CANRead_Std/3 -> Std_1/1
  CANRead_Std/4 -> Std_2/1
  CANRead_Std/5 -> Std_3/1
  Data Type ConversionStd/1 -> StdSelector_/1, StdSelector_1/1, StdSelector_2/1, StdSelector_3/1
  StdSelector_/1 -> StdStatus_/1
  StdSelector_1/1 -> StdStatus_1/1
  StdSelector_2/1 -> StdStatus_2/1
  StdSelector_3/1 -> StdStatus_3/1

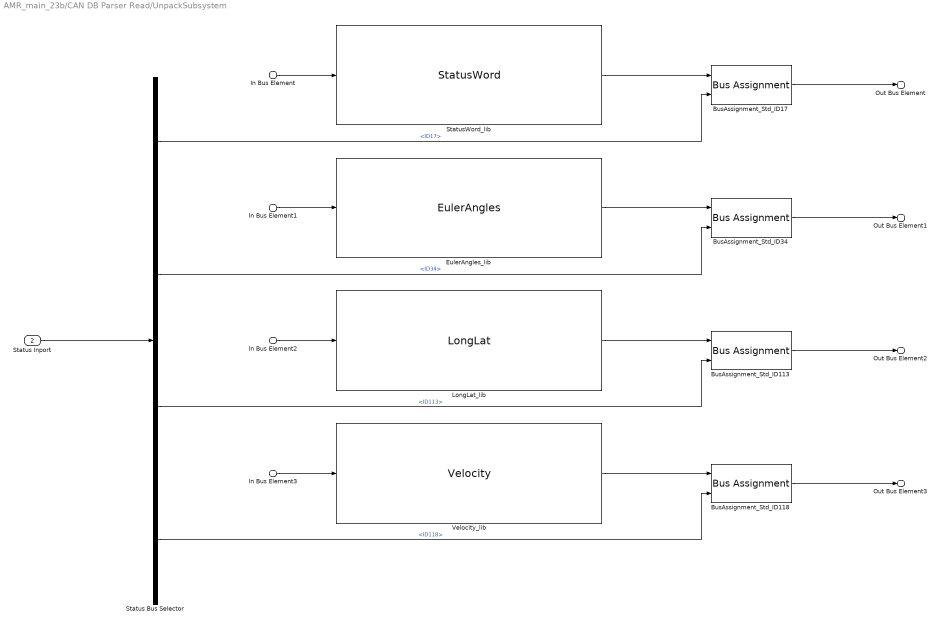
== system AMR_main_23b/CAN DB Parser Read/UnpackSubsystem ==
  In Bus Element : Inport  PortName=Unpack_In  Element=Std.ID17
  In Bus Element1 : Inport  PortName=Unpack_In  Element=Std.ID34
  In Bus Element2 : Inport  PortName=Unpack_In  Element=Std.ID113
  In Bus Element3 : Inport  PortName=Unpack_In  Element=Std.ID118
  Status Inport : Inport  Port=2
  BusAssignment_Std_ID{17,34,113,118} (4 alike) : BusAssignment  AssignedSignals=MessageStatus.Status
  EulerAngles_lib : tramontina_database_xsenslib/CAN unpack/EulerAngles  SystemSampleTime=-1  VariantActivationTime=update diagram  AllowFlexibleInterface=on  Latency=0  AutoFrameSizeCalculation=off
  LongLat_lib : tramontina_database_xsenslib/CAN unpack/LongLat  SystemSampleTime=-1  VariantActivationTime=update diagram  AllowFlexibleInterface=on  Latency=0  AutoFrameSizeCalculation=off
  Status Bus Selector : BusSelector  OutputSignals=Std.ID17,Std.ID34,Std.ID113,Std.ID118
  StatusWord_lib : tramontina_database_xsenslib/CAN unpack/StatusWord  SystemSampleTime=-1  VariantActivationTime=update diagram  AllowFlexibleInterface=on  Latency=0  AutoFrameSizeCalculation=off
  Velocity_lib : tramontina_database_xsenslib/CAN unpack/Velocity  SystemSampleTime=-1  VariantActivationTime=update diagram  AllowFlexibleInterface=on  Latency=0  AutoFrameSizeCalculation=off
  Out Bus Element : Outport  PortName=Unpack_Out  Element=ID17_StatusWord
  Out Bus Element1 : Outport  PortName=Unpack_Out  Element=ID34_EulerAngles
  Out Bus Element2 : Outport  PortName=Unpack_Out  Element=ID113_LongLat
  Out Bus Element3 : Outport  PortName=Unpack_Out  Element=ID118_Velocity
  wires:
  In Bus Element/1 -> StatusWord_lib/1
  StatusWord_lib/1 -> BusAssignment_Std_ID17/1
  BusAssignment_Std_ID17/1 -> Out Bus Element/1
  In Bus Element1/1 -> EulerAngles_lib/1
  EulerAngles_lib/1 -> BusAssignment_Std_ID34/1
  BusAssignment_Std_ID34/1 -> Out Bus Element1/1
  In Bus Element2/1 -> LongLat_lib/1
  LongLat_lib/1 -> BusAssignment_Std_ID113/1
  BusAssignment_Std_ID113/1 -> Out Bus Element2/1
  In Bus Element3/1 -> Velocity_lib/1
  Velocity_lib/1 -> BusAssignment_Std_ID118/1
  BusAssignment_Std_ID118/1 -> Out Bus Element3/1
  Status Inport/1 -> Status Bus Selector/1
  Status Bus Selector/1 -> BusAssignment_Std_ID17/2  "<ID17>"
  Status Bus Selector/2 -> BusAssignment_Std_ID34/2  "<ID34>"
  Status Bus Selector/3 -> BusAssignment_Std_ID113/2  "<ID113>"
  Status Bus Selector/4 -> BusAssignment_Std_ID118/2  "<ID118>"

== system AMR_main_23b/CAN DB Parser Read /ReadSubsystem ==
  CANRead_Std : speedgoatlib_IO60X_IO69X/CAN/CAN Read   moduleType=IO691  id=1  channel=1  canType=CAN (HS)  messageType=CAN (HS)  useBusOut=on  HasMulRead=Specify by IDs  MsgIDlist=[343]  isEFF=off  LabelInHex=off  enableInput=off  initValues=[691 1 0.05 0 1 1 0 1 2 0 1 343]  ts=50e-3
  Data Type ConversionStd : DataTypeConversion  OutDataTypeStr=uint8  SaturateOnIntegerOverflow=off  RndMeth=Floor
  StdSelector_ : Selector  IndexOptions=Index vector (dialog)  Indices=1  OutputSizes=1
  Std_ : Outport  PortName=Raw_Rx  Element=Std.ID343
  StdStatus_ : Outport  Port=2  PortName=Status_Rx  Element=Std.ID343
  wires:
  CANRead_Std/1 -> Data Type ConversionStd/1
  CANRead_Std/2 -> Std_/1
  Data Type ConversionStd/1 -> StdSelector_/1
  StdSelector_/1 -> StdStatus_/1

== system AMR_main_23b/CAN DB Parser Read /UnpackSubsystem ==
  In Bus Element : Inport  PortName=Unpack_In  Element=Std.ID343
  Status Inport : Inport  Port=2
  AMR_OperationMode_lib : tramontina_database_nvidialib/CAN unpack/AMR_OperationMode  SystemSampleTime=-1  VariantActivationTime=update diagram  AllowFlexibleInterface=on  Latency=0  AutoFrameSizeCalculation=off
  BusAssignment_Std_ID343 : BusAssignment  AssignedSignals=MessageStatus.Status
  Status Bus Selector : BusSelector  OutputSignals=Std.ID343
  Out Bus Element : Outport  PortName=Unpack_Out  Element=ID343_AMR_OperationMode
  wires:
  In Bus Element/1 -> AMR_OperationMode_lib/1
  AMR_OperationMode_lib/1 -> BusAssignment_Std_ID343/1
  BusAssignment_Std_ID343/1 -> Out Bus Element/1
  Status Inport/1 -> Status Bus Selector/1
  Status Bus Selector/1 -> BusAssignment_Std_ID343/2  "<ID343>"

== system AMR_main_23b/CAN DB Parser Read 1/ReadSubsystem ==
  CANRead_Std : speedgoatlib_IO60X_IO69X/CAN/CAN Read   moduleType=IO691  id=1  channel=1  canType=CAN (HS)  messageType=CAN (HS)  useBusOut=on  HasMulRead=Specify by IDs  MsgIDlist=[288]  isEFF=off  LabelInHex=off  enableInput=off  initValues=[691 1 0.005 0 1 1 0 1 2 0 1 288]  ts=5e-3
  Data Type ConversionStd : DataTypeConversion  OutDataTypeStr=uint8  SaturateOnIntegerOverflow=off  RndMeth=Floor
  StdSelector_ : Selector  IndexOptions=Index vector (dialog)  Indices=1  OutputSizes=1
  Std_ : Outport  PortName=Raw_Rx  Element=Std.ID288
  StdStatus_ : Outport  Port=2  PortName=Status_Rx  Element=Std.ID288
  wires:
  CANRead_Std/1 -> Data Type ConversionStd/1
  CANRead_Std/2 -> Std_/1
  Data Type ConversionStd/1 -> StdSelector_/1
  StdSelector_/1 -> StdStatus_/1

== system AMR_main_23b/CAN DB Parser Read 1/UnpackSubsystem ==
  In Bus Element : Inport  PortName=Unpack_In  Element=Std.ID288
  Status Inport : Inport  Port=2
  BusAssignment_Std_ID288 : BusAssignment  AssignedSignals=MessageStatus.Status
  Status Bus Selector : BusSelector  OutputSignals=Std.ID288
  mobotic_feedback_pos_lib : tramontina_database_nvidialib/CAN unpack/mobotic_feedback_pos  SystemSampleTime=-1  VariantActivationTime=update diagram  AllowFlexibleInterface=on  Latency=0  AutoFrameSizeCalculation=off
  Out Bus Element : Outport  PortName=Unpack_Out  Element=ID288_mobotic_feedback_pos
  wires:
  In Bus Element/1 -> mobotic_feedback_pos_lib/1
  mobotic_feedback_pos_lib/1 -> BusAssignment_Std_ID288/1
  BusAssignment_Std_ID288/1 -> Out Bus Element/1
  Status Inport/1 -> Status Bus Selector/1
  Status Bus Selector/1 -> BusAssignment_Std_ID288/2  "<ID288>"

== system AMR_main_23b/CAN DB Parser Read 2/ReadSubsystem ==
  CANRead_Std : speedgoatlib_IO60X_IO69X/CAN/CAN Read   moduleType=IO691  id=1  channel=1  canType=CAN (HS)  messageType=CAN (HS)  useBusOut=on  HasMulRead=Specify by IDs  MsgIDlist="[422  423]"  isEFF=off  LabelInHex=off  enableInput=off  initValues=[691 1 0.05 0 1 1 0 1 2 0 2 422 423]  ts=50e-3
  Data Type ConversionStd : DataTypeConversion  OutDataTypeStr=uint8  SaturateOnIntegerOverflow=off  RndMeth=Floor
  StdSelector_ : Selector  IndexOptions=Index vector (dialog)  Indices=1  OutputSizes=1
  StdSelector_1 : Selector  IndexOptions=Index vector (dialog)  Indices=2  OutputSizes=1
  Std_ : Outport  PortName=Raw_Rx  Element=Std.ID422
  Std_1 : Outport  PortName=Raw_Rx  Element=Std.ID423
  StdStatus_ : Outport  Port=2  PortName=Status_Rx  Element=Std.ID422
  StdStatus_1 : Outport  Port=2  PortName=Status_Rx  Element=Std.ID423
  wires:
  CANRead_Std/1 -> Data Type ConversionStd/1
  CANRead_Std/2 -> Std_/1
  CANRead_Std/3 -> Std_1/1
  Data Type ConversionStd/1 -> StdSelector_/1, StdSelector_1/1
  StdSelector_/1 -> StdStatus_/1
  StdSelector_1/1 -> StdStatus_1/1

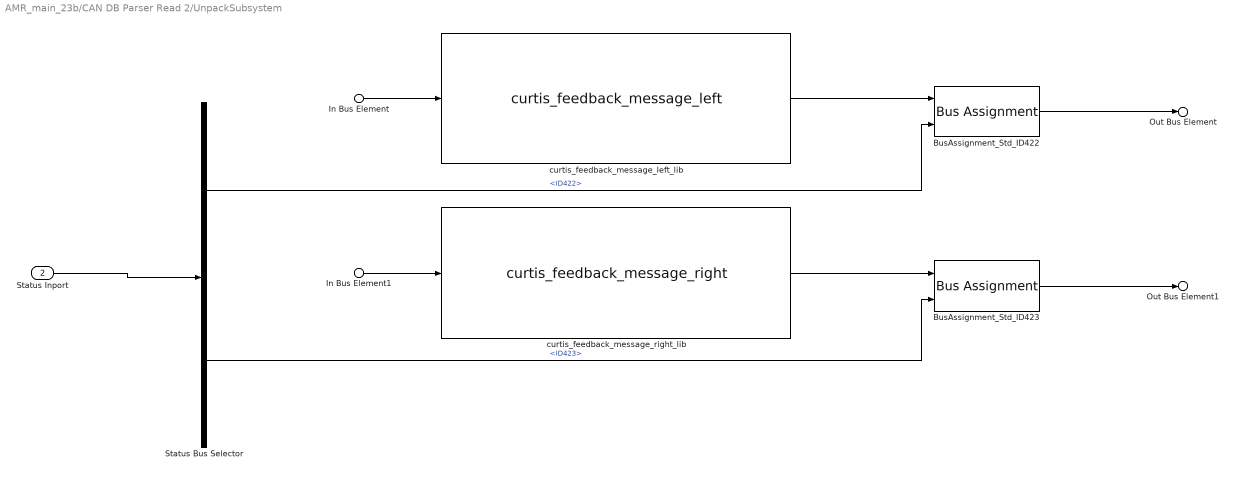
== system AMR_main_23b/CAN DB Parser Read 2/UnpackSubsystem ==
  In Bus Element : Inport  PortName=Unpack_In  Element=Std.ID422
  In Bus Element1 : Inport  PortName=Unpack_In  Element=Std.ID423
  Status Inport : Inport  Port=2
  BusAssignment_Std_ID422 : BusAssignment  AssignedSignals=MessageStatus.Status
  BusAssignment_Std_ID423 : BusAssignment  AssignedSignals=MessageStatus.Status
  Status Bus Selector : BusSelector  OutputSignals=Std.ID422,Std.ID423
  curtis_feedback_message_left_lib : tramontina_database_curtislib/CAN unpack/curtis_feedback_message_left  SystemSampleTime=-1  VariantActivationTime=update diagram  AllowFlexibleInterface=on  Latency=0  AutoFrameSizeCalculation=off
  curtis_feedback_message_right_lib : tramontina_database_curtislib/CAN unpack/curtis_feedback_message_right  SystemSampleTime=-1  VariantActivationTime=update diagram  AllowFlexibleInterface=on  Latency=0  AutoFrameSizeCalculation=off
  Out Bus Element : Outport  PortName=Unpack_Out  Element=ID422_curtis_feedback_message_left
  Out Bus Element1 : Outport  PortName=Unpack_Out  Element=ID423_curtis_feedback_message_right
  wires:
  In Bus Element/1 -> curtis_feedback_message_left_lib/1
  curtis_feedback_message_left_lib/1 -> BusAssignment_Std_ID422/1
  BusAssignment_Std_ID422/1 -> Out Bus Element/1
  In Bus Element1/1 -> curtis_feedback_message_right_lib/1
  curtis_feedback_message_right_lib/1 -> BusAssignment_Std_ID423/1
  BusAssignment_Std_ID423/1 -> Out Bus Element1/1
  Status Inport/1 -> Status Bus Selector/1
  Status Bus Selector/1 -> BusAssignment_Std_ID422/2  "<ID422>"
  Status Bus Selector/2 -> BusAssignment_Std_ID423/2  "<ID423>"

== system AMR_main_23b/CAN DB Parser Read 3/ReadSubsystem ==
  CANRead_Std : speedgoatlib_IO60X_IO69X/CAN/CAN Read   moduleType=IO691  id=1  channel=1  canType=CAN (HS)  messageType=CAN (HS)  useBusOut=on  HasMulRead=Specify by IDs  MsgIDlist="[1830  1831]"  isEFF=off  LabelInHex=off  enableInput=off  initValues=[691 1 0.5 0 1 1 0 1 2 0 2 1830 1831]  ts=500e-3
  Data Type ConversionStd : DataTypeConversion  OutDataTypeStr=uint8  SaturateOnIntegerOverflow=off  RndMeth=Floor
  StdSelector_ : Selector  IndexOptions=Index vector (dialog)  Indices=1  OutputSizes=1
  StdSelector_1 : Selector  IndexOptions=Index vector (dialog)  Indices=2  OutputSizes=1
  Std_ : Outport  PortName=Raw_Rx  Element=Std.ID1830
  Std_1 : Outport  PortName=Raw_Rx  Element=Std.ID1831
  StdStatus_ : Outport  Port=2  PortName=Status_Rx  Element=Std.ID1830
  StdStatus_1 : Outport  Port=2  PortName=Status_Rx  Element=Std.ID1831
  wires:
  CANRead_Std/1 -> Data Type ConversionStd/1
  CANRead_Std/2 -> Std_/1
  CANRead_Std/3 -> Std_1/1
  Data Type ConversionStd/1 -> StdSelector_/1, StdSelector_1/1
  StdSelector_/1 -> StdStatus_/1
  StdSelector_1/1 -> StdStatus_1/1

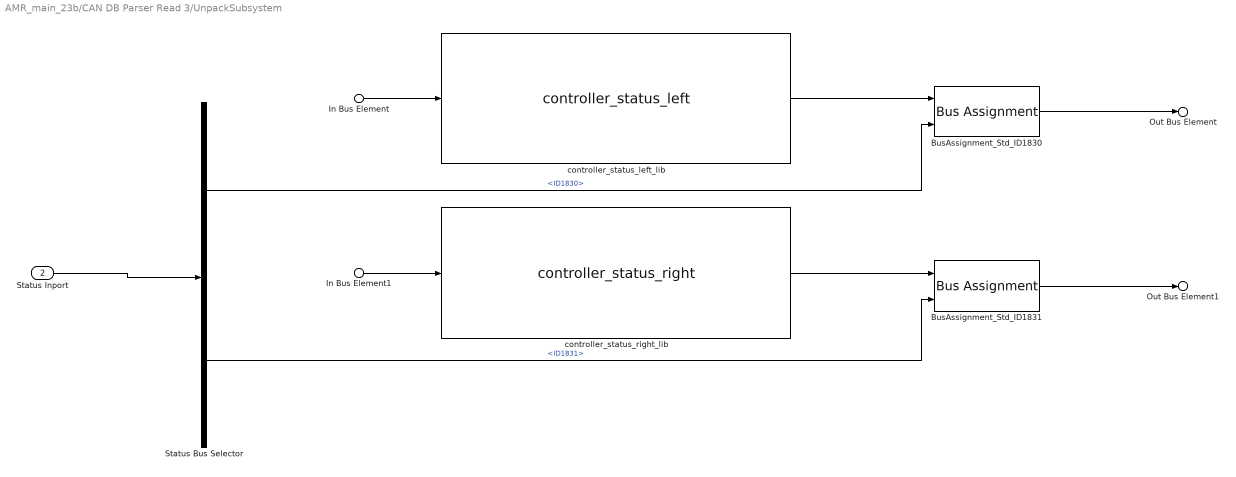
== system AMR_main_23b/CAN DB Parser Read 3/UnpackSubsystem ==
  In Bus Element : Inport  PortName=Unpack_In  Element=Std.ID1830
  In Bus Element1 : Inport  PortName=Unpack_In  Element=Std.ID1831
  Status Inport : Inport  Port=2
  BusAssignment_Std_ID1830 : BusAssignment  AssignedSignals=MessageStatus.Status
  BusAssignment_Std_ID1831 : BusAssignment  AssignedSignals=MessageStatus.Status
  Status Bus Selector : BusSelector  OutputSignals=Std.ID1830,Std.ID1831
  controller_status_left_lib : tramontina_database_curtislib/CAN unpack/controller_status_left  SystemSampleTime=-1  VariantActivationTime=update diagram  AllowFlexibleInterface=on  Latency=0  AutoFrameSizeCalculation=off
  controller_status_right_lib : tramontina_database_curtislib/CAN unpack/controller_status_right  SystemSampleTime=-1  VariantActivationTime=update diagram  AllowFlexibleInterface=on  Latency=0  AutoFrameSizeCalculation=off
  Out Bus Element : Outport  PortName=Unpack_Out  Element=ID1830_controller_status_left
  Out Bus Element1 : Outport  PortName=Unpack_Out  Element=ID1831_controller_status_right
  wires:
  In Bus Element/1 -> controller_status_left_lib/1
  controller_status_left_lib/1 -> BusAssignment_Std_ID1830/1
  BusAssignment_Std_ID1830/1 -> Out Bus Element/1
  In Bus Element1/1 -> controller_status_right_lib/1
  controller_status_right_lib/1 -> BusAssignment_Std_ID1831/1
  BusAssignment_Std_ID1831/1 -> Out Bus Element1/1
  Status Inport/1 -> Status Bus Selector/1
  Status Bus Selector/1 -> BusAssignment_Std_ID1830/2  "<ID1830>"
  Status Bus Selector/2 -> BusAssignment_Std_ID1831/2  "<ID1831>"

== system AMR_main_23b/CAN DB Parser Read 4/ReadSubsystem ==
  CANRead_Std : speedgoatlib_IO60X_IO69X/CAN/CAN Read   moduleType=IO691  id=1  channel=1  canType=CAN (HS)  messageType=CAN (HS)  useBusOut=on  HasMulRead=Specify by IDs  MsgIDlist=[341]  isEFF=off  LabelInHex=off  enableInput=off  initValues=[691 1 0.1 0 1 1 0 1 2 0 1 341]  ts=100e-3
  Data Type ConversionStd : DataTypeConversion  OutDataTypeStr=uint8  SaturateOnIntegerOverflow=off  RndMeth=Floor
  StdSelector_ : Selector  IndexOptions=Index vector (dialog)  Indices=1  OutputSizes=1
  Std_ : Outport  PortName=Raw_Rx  Element=Std.ID341
  StdStatus_ : Outport  Port=2  PortName=Status_Rx  Element=Std.ID341
  wires:
  CANRead_Std/1 -> Data Type ConversionStd/1
  CANRead_Std/2 -> Std_/1
  Data Type ConversionStd/1 -> StdSelector_/1
  StdSelector_/1 -> StdStatus_/1

== system AMR_main_23b/CAN DB Parser Read 4/UnpackSubsystem ==
  In Bus Element : Inport  PortName=Unpack_In  Element=Std.ID341
  Status Inport : Inport  Port=2
  BusAssignment_Std_ID341 : BusAssignment  AssignedSignals=MessageStatus.Status
  Status Bus Selector : BusSelector  OutputSignals=Std.ID341
  read_from_flexisoft_lib : tramontina_database_sick_modbuslib/CAN unpack/read_from_flexisoft  SystemSampleTime=-1  VariantActivationTime=update diagram  AllowFlexibleInterface=on  Latency=0  AutoFrameSizeCalculation=off
  Out Bus Element : Outport  PortName=Unpack_Out  Element=ID341_read_from_flexisoft
  wires:
  In Bus Element/1 -> read_from_flexisoft_lib/1
  read_from_flexisoft_lib/1 -> BusAssignment_Std_ID341/1
  BusAssignment_Std_ID341/1 -> Out Bus Element/1
  Status Inport/1 -> Status Bus Selector/1
  Status Bus Selector/1 -> BusAssignment_Std_ID341/2  "<ID341>"

== system AMR_main_23b/CAN DB Parser Read 5/ReadSubsystem ==
  CANRead_Std : speedgoatlib_IO60X_IO69X/CAN/CAN Read   moduleType=IO691  id=1  channel=1  canType=CAN (HS)  messageType=CAN (HS)  useBusOut=on  HasMulRead=Specify by IDs  MsgIDlist="[368  369]"  isEFF=off  LabelInHex=off  enableInput=off  initValues=[691 1 0.01 0 1 1 0 1 2 0 2 368 369]  ts=10e-3
  Data Type ConversionStd : DataTypeConversion  OutDataTypeStr=uint8  SaturateOnIntegerOverflow=off  RndMeth=Floor
  StdSelector_ : Selector  IndexOptions=Index vector (dialog)  Indices=1  OutputSizes=1
  StdSelector_1 : Selector  IndexOptions=Index vector (dialog)  Indices=2  OutputSizes=1
  Std_ : Outport  PortName=Raw_Rx  Element=Std.ID368
  Std_1 : Outport  PortName=Raw_Rx  Element=Std.ID369
  StdStatus_ : Outport  Port=2  PortName=Status_Rx  Element=Std.ID368
  StdStatus_1 : Outport  Port=2  PortName=Status_Rx  Element=Std.ID369
  wires:
  CANRead_Std/1 -> Data Type ConversionStd/1
  CANRead_Std/2 -> Std_/1
  CANRead_Std/3 -> Std_1/1
  Data Type ConversionStd/1 -> StdSelector_/1, StdSelector_1/1
  StdSelector_/1 -> StdStatus_/1
  StdSelector_1/1 -> StdStatus_1/1
